simulink model "motor_rotacao"  (R2025b)
settings: Solver=VariableStepAuto  StartTime=0.0  StopTime=10  RelTol=1e-3
values from neighbouring files (symbols this model uses):
  J = 0.25    [parametros.m]
  RPM = 800    [parametros.m]
settings Model: Creator=thiag  LastModifiedBy=thiag

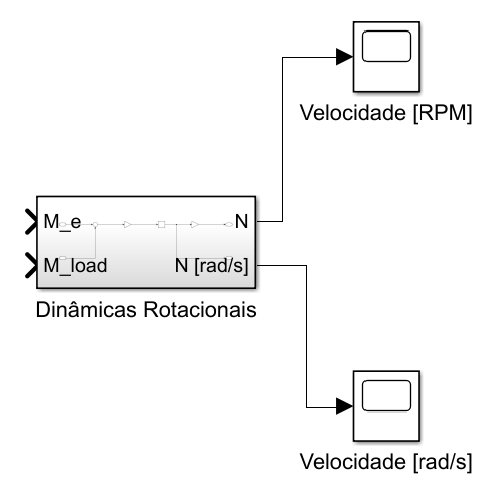
[thumbnail: Simulink's stored preview of the top-level diagram]
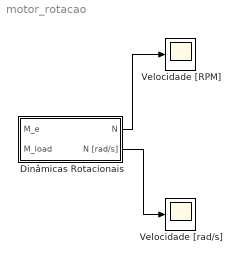
== system motor_rotacao ==
  Dinâmicas Rotacionais : Subsystem
  Velocidade [RPM] : Scope
      settings: ActiveDisplayYMinimum=-125.55980551817186  ActiveDisplayYMaximum=7646.8825914479748
  Velocidade [rad/s] : Scope
      settings: ActiveDisplayYMinimum=-166.22419590427216  ActiveDisplayYMaximum=2333.7758040957283
  wires:
  Dinâmicas Rotacionais/1(N) -> Velocidade [RPM]/1
  Dinâmicas Rotacionais/2(N [rad/s]) -> Velocidade [rad/s]/1

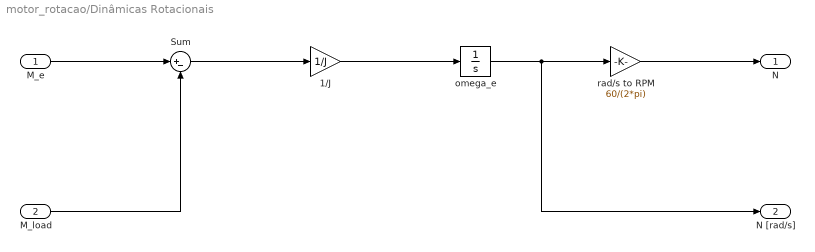
== system motor_rotacao/Dinâmicas Rotacionais ==
  M_e : Inport
  M_load : Inport  Port=2
  1/J : Gain  Gain=1/J
  Sum : Sum  Inputs=|+-
  omega_e : Integrator  InitialCondition=(RPM*2*pi)/60
  rad/s to RPM : Gain  Gain=60/(2*pi)
  N : Outport
  N [rad/s] : Outport  Port=2
  wires:
  M_e/1 -> Sum/1
  M_load/1 -> Sum/2
  Sum/1 -> 1/J/1
  1/J/1 -> omega_e/1
  omega_e/1 -> N [rad/s]/1, rad/s to RPM/1
  rad/s to RPM/1 -> N/1
